simulink model "comm_test"  (R2022a)
settings: Solver=FixedStepAuto  StartTime=0.0  StopTime=20  RelTol=1e-3
libraries: hdlsllib x8, simulink x7, mbedblockslib x7
settings Model: ExtModeTrigDuration=10  Creator=FUGAZI  LastModifiedBy=FUGAZI
settings OptimizationCC: EnhancedBackFolding=on  PassReuseOutputArgsAs=Individual arguments  ZeroExternalMemoryAtStartup=off  ZeroInternalMemoryAtStartup=off  MaxStackSize=64  OptimizeBlockOrder=speed  DifferentSizesBufferReuse=on  OptimizationCustomize=off  EfficientTunableParamExpr=on
settings DebuggingCC: ParameterTunabilityLossMsg=error
settings HardwareCC: ProdBitPerPointer=32  ProdBitPerSizeT=32  ProdBitPerPtrDiffT=32  ProdLargestAtomicInteger=Long  ProdLargestAtomicFloat=Double  ProdWordSize=32  ProdLongLongMode=on  ProdHWDeviceType=ARM Compatible->ARM Cortex
settings SFSimCC: MATLABDynamicMemAlloc=off
settings RTWCC: SystemTargetFile=ert.tlc  HardwareBoard=STM32 Nucleo L476RG  TemplateMakefile=ert_default_tmf  Toolchain=GNU Tools for ARM Embedded Processors
settings CodeAppCC: ForceParamTrailComments=on  IgnoreCustomStorageClasses=off  OperatorAnnotations=on  SimulinkDataObjDesc=on  SFDataObjDesc=on  InsertBlockDesc=on
settings ERTTargetCC: ExtModeTransport=3  ExtModeStaticAlloc=on  ExtModeStaticAllocSize=2000  ExtModeMexFile=ext_xcp  ExtModeIntrfLevel=Level2 - Open

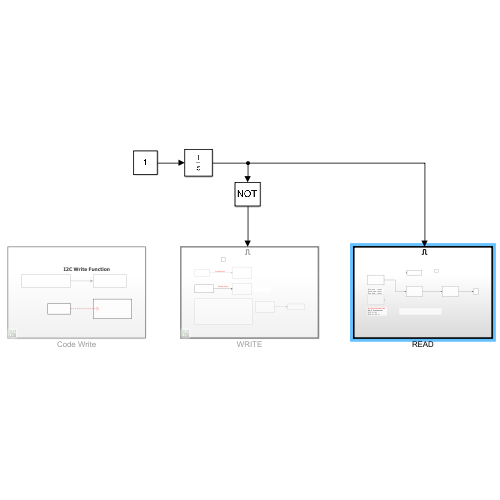
[thumbnail: Simulink's stored preview of the top-level diagram]
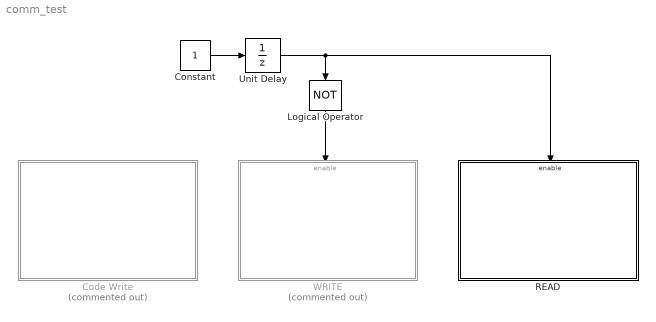
== system comm_test ==
  Code Write : Subsystem  Commented=on
  Constant : Constant  OutDataTypeStr=boolean  SampleTime=0.1
  Logical Operator : Logic  Operator=NOT  AllPortsSameDT=off  OutDataTypeStr=boolean
  READ : Subsystem
  Unit Delay : UnitDelay  SampleTime=-1  HasFrameUpgradeWarning=on
  WRITE : Subsystem  Commented=on
  wires:
  Constant/1 -> Unit Delay/1
  Logical Operator/1 -> WRITE/Enable
  Unit Delay/1 -> READ/Enable, Logical Operator/1

== system comm_test/Code Write ==
  note: I2C Write Function
  Constant : Constant  Value=[0x10, 0x00]
  Constant1 : Constant  Commented=on  Value=[hex2dec('20'), hex2dec('51')]
  Display : Display  Commented=on
  MATLAB Function : MATLAB Function  TreatAsAtomicUnit=on
  wires:
  Constant/1 -> ?
  Constant1/1 -> Display/1

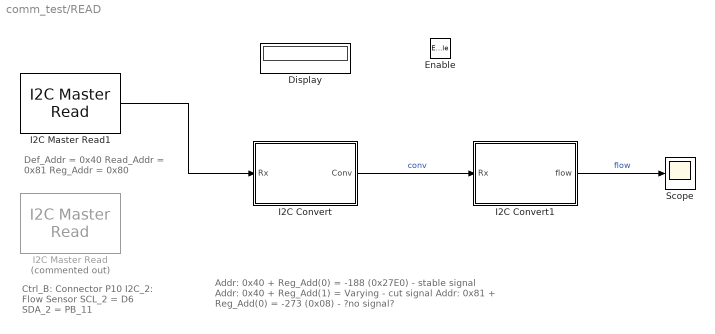
== system comm_test/READ ==
  note: Def_Addr = 0x40
      | Read_Addr = 0x81
      | Reg_Addr = 0x80
  note: Ctrl_B: Connector P10
      | I2C_2: Flow Sensor
      | SCL_2 = D6
      | SDA_2 = PB_11
  note: Addr: 0x40  + Reg_Add(0) = -188 (0x27E0) - stable signal
      | Addr: 0x40  + Reg_Add(1) = Varying            - cut signal
      | Addr: 0x81  + Reg_Add(0) = -273 (0x08)	     - ?no signal?
  Enable : EnablePort
  Display : Display
  I2C Convert : Subsystem
  I2C Convert1 : Subsystem
  I2C Master Read : mbedblockslib/I2C Master Read  Commented=on  I2CModule=0  Mode=Master  SlaveAddress=hex2dec('81')  SlaveByteOrder=BigEndian  Direction=Receiver  RegisterAddressMode=on  RegisterAddress=uint8(0)  SlaveDataType=uint8  DataLength=3  NoAck=off  RepeatedStart=on  OutputStatus=off  SampleTime=0.1
      settings: SourceProductBaseCode=MICROBIT,NUCLEO,STMICRODIS
  I2C Master Read1 : mbedblockslib/I2C Master Read  I2CModule=0  Mode=Master  SlaveAddress=hex2dec('40')  SlaveByteOrder=BigEndian  Direction=Receiver  RegisterAddressMode=off  RegisterAddress=uint8(1)  SlaveDataType=uint8  DataLength=3  NoAck=off  RepeatedStart=off  OutputStatus=off  SampleTime=0.5
      settings: SourceProductBaseCode=MICROBIT,NUCLEO,STMICRODIS
  Scope : Scope
  wires:
  I2C Convert1/1(flow) -> Scope/1  "flow"
  I2C Master Read1/1 -> I2C Convert/1(Rx)
  I2C Convert/1(Conv) -> I2C Convert1/1(Rx)  "conv"

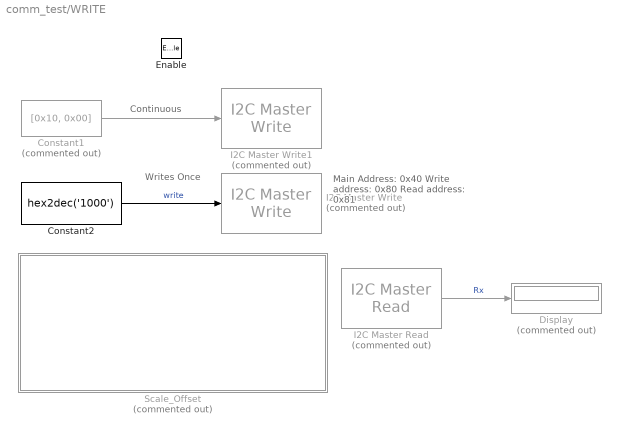
== system comm_test/WRITE ==
  note: Writes Once
  note: Main Address: 0x40
      | Write address: 0x80
      | Read address: 0x81
  note: Continuous
  Enable : EnablePort
  Constant1 : Constant  Commented=on  Value=[0x10, 0x00]
  Constant2 : Constant  Value=hex2dec('1000')  OutDataTypeStr=uint16
  Display : Display  Commented=on
  I2C Master Read : mbedblockslib/I2C Master Read  Commented=on  I2CModule=0  Mode=Master  SlaveAddress=hex2dec('40')  SlaveByteOrder=BigEndian  Direction=Receiver  RegisterAddressMode=on  RegisterAddress=uint8(1)  SlaveDataType=uint8  DataLength=3  NoAck=off  RepeatedStart=on  OutputStatus=off  SampleTime=0.1
      settings: SourceProductBaseCode=MICROBIT,NUCLEO,STMICRODIS
  I2C Master Write : mbedblockslib/I2C Master Write  Commented=on  I2CModule=0  Mode=Master  SlaveAddress=hex2dec('40')  SlaveByteOrder=BigEndian  Direction=Transmitter  RegisterAddressMode=on  RegisterAddress=uint8(1)  SlaveDataType=uint8  DataLength=2  NoAck=off  RepeatedStart=on  OutputStatus=off
      settings: SourceProductBaseCode=MICROBIT,NUCLEO,STMICRODIS
  I2C Master Write1 : mbedblockslib/I2C Master Write  Commented=on  I2CModule=0  Mode=Master  SlaveAddress=hex2dec('40')  SlaveByteOrder=BigEndian  Direction=Transmitter  RegisterAddressMode=on  RegisterAddress=uint8(1)  SlaveDataType=uint8  DataLength=2  NoAck=off  RepeatedStart=on  OutputStatus=off
      settings: SourceProductBaseCode=MICROBIT,NUCLEO,STMICRODIS
  Scale_Offset : Subsystem  Commented=on
  wires:
  Constant2/1 -> I2C Master Write/1  "write"
  Constant1/1 -> I2C Master Write1/1
  I2C Master Read/1 -> Display/1  "Rx"

== system comm_test/READ/I2C Convert ==
  note: Possible Range:
      | 0x0666 = -xx SLM
      | 0x1FF7 = 0 SLM
      | 0x3999 = xx SLM
  note: Flow Rate Range: 10sL/m - 80sL/m
  note: I2C:
      | * 1 byte @ 16-bit
      | * 2 byte @ 8-bit
      | * 3 byte @ 8-bit
      | * 4 byte @ 8-bit
  note: Add 3rd byte for CRC?
  Rx : Inport
  (2x) 8-bit : Subsystem  Commented=on
  (3x) 8-bit : Subsystem
  (4x) 8-bit : Subsystem  Commented=on
  Conv : Outport
  wires:
  Rx/1 -> (3x) 8-bit/1(Rx)  "Rx"
  (3x) 8-bit/1(3-byte) -> Conv/1  "3_byte"

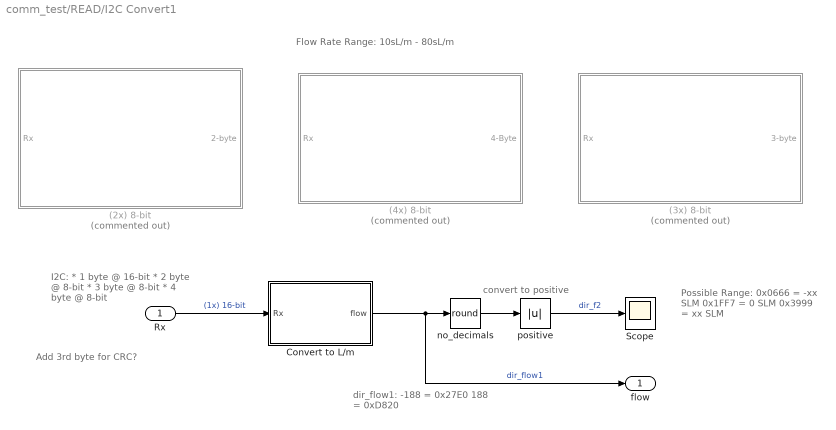
== system comm_test/READ/I2C Convert1 ==
  note: dir_flow1:
      | -188 = 0x27E0
      | 188 = 0xD820
  note: Possible Range:
      | 0x0666 = -xx SLM
      | 0x1FF7 = 0 SLM
      | 0x3999 = xx SLM
  note: Flow Rate Range: 10sL/m - 80sL/m
  note: I2C:
      | * 1 byte @ 16-bit
      | * 2 byte @ 8-bit
      | * 3 byte @ 8-bit
      | * 4 byte @ 8-bit
  note: Add 3rd byte for CRC?
  note: convert to positive
  Rx : Inport
  (2x) 8-bit : Subsystem  Commented=on
  (3x) 8-bit : Subsystem  Commented=on
  (4x) 8-bit : Subsystem  Commented=on
  Convert to L/m : Subsystem
  Scope : Scope
  no_decimals : Rounding  Operator=round
  positive : Abs  SaturateOnIntegerOverflow=off
  flow : Outport
  wires:
  Convert to L/m/1(flow) -> flow/1, no_decimals/1  "dir_flow1"
  no_decimals/1 -> positive/1
  Rx/1 -> Convert to L/m/1(Rx)  "(1x) 16-bit"
  positive/1 -> Scope/1  "dir_f2"

== system comm_test/WRITE/Scale_Offset ==
  note: Should be ~0.5ms between writes
  Constant3 : Constant  Value=[hex2dec('31E3'), hex2dec('31E4')]  OutDataTypeStr=uint16
  Display : Display  Commented=on
      settings: Format=hex (Stored Integer)
  Display1 : Display
      settings: Format=hex (Stored Integer)
  I2C Master Read : mbedblockslib/I2C Master Read  I2CModule=0  Mode=Master  SlaveAddress=hex2dec('40')  SlaveByteOrder=BigEndian  Direction=Receiver  RegisterAddressMode=on  RegisterAddress=uint8(1)  SlaveDataType=uint16  DataLength=1  NoAck=off  RepeatedStart=off  OutputStatus=off  SampleTime=0.1
      settings: SourceProductBaseCode=MICROBIT,NUCLEO,STMICRODIS
  I2C Master Write2 : mbedblockslib/I2C Master Write  I2CModule=0  Mode=Master  SlaveAddress=hex2dec('40')  SlaveByteOrder=BigEndian  Direction=Transmitter  RegisterAddressMode=on  RegisterAddress=uint8(1)  SlaveDataType=uint8  DataLength=2  NoAck=off  RepeatedStart=on  OutputStatus=off
      settings: SourceProductBaseCode=MICROBIT,NUCLEO,STMICRODIS
  wires:
  Constant3/1 -> I2C Master Write2/1, Display/1  "offset_scale"
  I2C Master Read/1 -> Display1/1  "read"

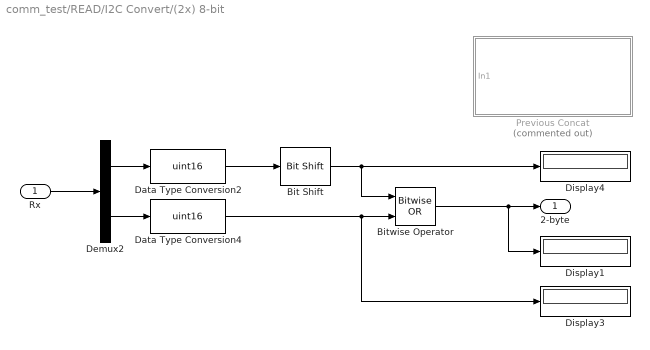
== system comm_test/READ/I2C Convert/(2x) 8-bit ==
  Rx : Inport
  Bit Shift : hdlsllib/Logic and Bit Operations/Bit Shift  mode=Shift Left Logical  N=8
  Bitwise Operator : simulink/Logic and Bit Operations/Bitwise Operator  logicop=OR  UseBitMask=off  NumInputPorts=2  BitMask=bin2dec('11011001')  BitMaskRealWorld=Stored Integer
  Data Type Conversion2 : DataTypeConversion  OutDataTypeStr=uint16  SaturateOnIntegerOverflow=off  RndMeth=Floor
  Data Type Conversion4 : DataTypeConversion  OutDataTypeStr=uint16  SaturateOnIntegerOverflow=off  RndMeth=Floor
  Demux2 : Demux  Outputs=2
  Display1 : Display
      settings: Format=hex (Stored Integer)
  Display3 : Display
      settings: Format=hex (Stored Integer)
  Display4 : Display
      settings: Format=hex (Stored Integer)
  Previous Concat : Subsystem  Commented=on
  2-byte : Outport
  wires:
  Rx/1 -> Demux2/1
  Demux2/1 -> Data Type Conversion2/1
  Data Type Conversion2/1 -> Bit Shift/1
  Bit Shift/1 -> Display4/1, Bitwise Operator/1
  Data Type Conversion4/1 -> Display3/1, Bitwise Operator/2
  Demux2/2 -> Data Type Conversion4/1
  Bitwise Operator/1 -> Display1/1, 2-byte/1

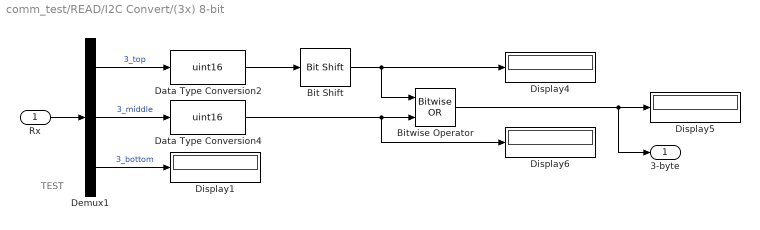
== system comm_test/READ/I2C Convert/(3x) 8-bit ==
  note: TEST
  Rx : Inport
  Bit Shift : hdlsllib/Logic and Bit Operations/Bit Shift  mode=Shift Left Logical  N=8
  Bitwise Operator : simulink/Logic and Bit Operations/Bitwise Operator  logicop=OR  UseBitMask=off  NumInputPorts=2  BitMask=bin2dec('11011001')  BitMaskRealWorld=Stored Integer
  Data Type Conversion2 : DataTypeConversion  OutDataTypeStr=uint16  SaturateOnIntegerOverflow=off  RndMeth=Floor
  Data Type Conversion4 : DataTypeConversion  OutDataTypeStr=uint16  SaturateOnIntegerOverflow=off  RndMeth=Floor
  Demux1 : Demux  Outputs=3
  Display{1,4..6} (4 alike) : Display
      settings: Format=hex (Stored Integer)
  3-byte : Outport
  wires:
  Bit Shift/1 -> Bitwise Operator/1, Display4/1
  Data Type Conversion4/1 -> Display6/1, Bitwise Operator/2
  Bitwise Operator/1 -> 3-byte/1, Display5/1
  Data Type Conversion2/1 -> Bit Shift/1
  Rx/1 -> Demux1/1
  Demux1/1 -> Data Type Conversion2/1  "3_top"
  Demux1/2 -> Data Type Conversion4/1  "3_middle"
  Demux1/3 -> Display1/1  "3_bottom"

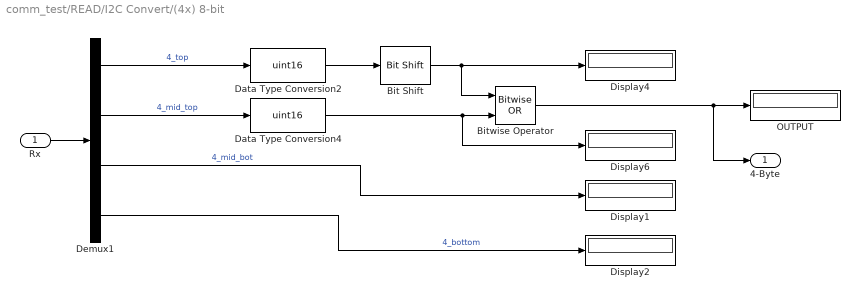
== system comm_test/READ/I2C Convert/(4x) 8-bit ==
  Rx : Inport
  Bit Shift : hdlsllib/Logic and Bit Operations/Bit Shift  mode=Shift Left Logical  N=8
  Bitwise Operator : simulink/Logic and Bit Operations/Bitwise Operator  logicop=OR  UseBitMask=off  NumInputPorts=2  BitMask=bin2dec('11011001')  BitMaskRealWorld=Stored Integer
  Data Type Conversion2 : DataTypeConversion  OutDataTypeStr=uint16  SaturateOnIntegerOverflow=off  RndMeth=Floor
  Data Type Conversion4 : DataTypeConversion  OutDataTypeStr=uint16  SaturateOnIntegerOverflow=off  RndMeth=Floor
  Demux1 : Demux
  Display{1..2,4,6} (4 alike) : Display
      settings: Format=hex (Stored Integer)
  OUTPUT : Display
      settings: Format=hex (Stored Integer)
  4-Byte : Outport
  wires:
  Data Type Conversion2/1 -> Bit Shift/1
  Bitwise Operator/1 -> 4-Byte/1, OUTPUT/1
  Bit Shift/1 -> Display4/1, Bitwise Operator/1
  Demux1/4 -> Display2/1  "4_bottom"
  Rx/1 -> Demux1/1
  Demux1/2 -> Data Type Conversion4/1  "4_mid_top"
  Demux1/1 -> Data Type Conversion2/1  "4_top"
  Data Type Conversion4/1 -> Display6/1, Bitwise Operator/2
  Demux1/3 -> Display1/1  "4_mid_bot"

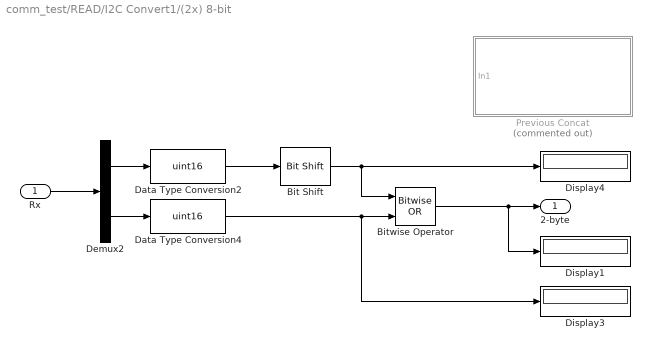
== system comm_test/READ/I2C Convert1/(2x) 8-bit ==
  Rx : Inport
  Bit Shift : hdlsllib/Logic and Bit Operations/Bit Shift  mode=Shift Left Logical  N=8
  Bitwise Operator : simulink/Logic and Bit Operations/Bitwise Operator  logicop=OR  UseBitMask=off  NumInputPorts=2  BitMask=bin2dec('11011001')  BitMaskRealWorld=Stored Integer
  Data Type Conversion2 : DataTypeConversion  OutDataTypeStr=uint16  SaturateOnIntegerOverflow=off  RndMeth=Floor
  Data Type Conversion4 : DataTypeConversion  OutDataTypeStr=uint16  SaturateOnIntegerOverflow=off  RndMeth=Floor
  Demux2 : Demux  Outputs=2
  Display1 : Display
      settings: Format=hex (Stored Integer)
  Display3 : Display
      settings: Format=hex (Stored Integer)
  Display4 : Display
      settings: Format=hex (Stored Integer)
  Previous Concat : Subsystem  Commented=on
  2-byte : Outport
  wires:
  Rx/1 -> Demux2/1
  Demux2/1 -> Data Type Conversion2/1
  Data Type Conversion2/1 -> Bit Shift/1
  Bit Shift/1 -> Display4/1, Bitwise Operator/1
  Data Type Conversion4/1 -> Display3/1, Bitwise Operator/2
  Demux2/2 -> Data Type Conversion4/1
  Bitwise Operator/1 -> Display1/1, 2-byte/1

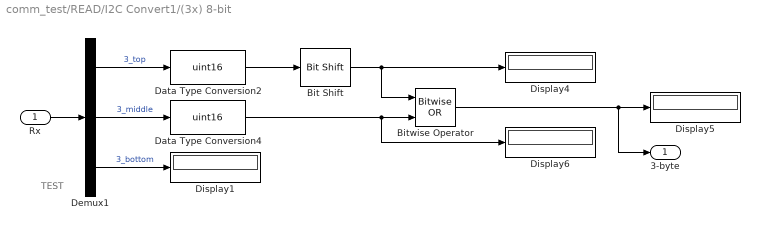
== system comm_test/READ/I2C Convert1/(3x) 8-bit ==
  note: TEST
  Rx : Inport
  Bit Shift : hdlsllib/Logic and Bit Operations/Bit Shift  mode=Shift Left Logical  N=8
  Bitwise Operator : simulink/Logic and Bit Operations/Bitwise Operator  logicop=OR  UseBitMask=off  NumInputPorts=2  BitMask=bin2dec('11011001')  BitMaskRealWorld=Stored Integer
  Data Type Conversion2 : DataTypeConversion  OutDataTypeStr=uint16  SaturateOnIntegerOverflow=off  RndMeth=Floor
  Data Type Conversion4 : DataTypeConversion  OutDataTypeStr=uint16  SaturateOnIntegerOverflow=off  RndMeth=Floor
  Demux1 : Demux  Outputs=3
  Display{1,4..6} (4 alike) : Display
      settings: Format=hex (Stored Integer)
  3-byte : Outport
  wires:
  Bit Shift/1 -> Bitwise Operator/1, Display4/1
  Data Type Conversion4/1 -> Display6/1, Bitwise Operator/2
  Bitwise Operator/1 -> 3-byte/1, Display5/1
  Data Type Conversion2/1 -> Bit Shift/1
  Rx/1 -> Demux1/1
  Demux1/1 -> Data Type Conversion2/1  "3_top"
  Demux1/2 -> Data Type Conversion4/1  "3_middle"
  Demux1/3 -> Display1/1  "3_bottom"

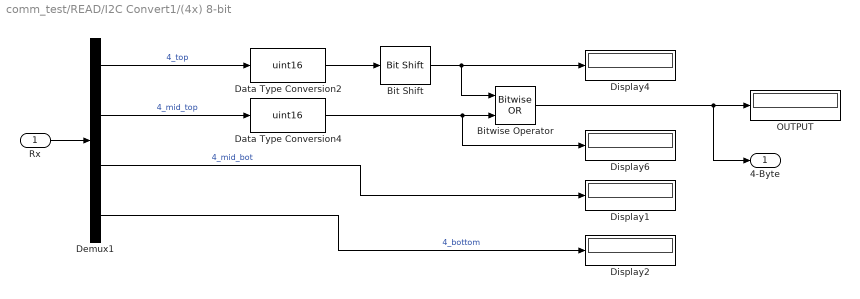
== system comm_test/READ/I2C Convert1/(4x) 8-bit ==
  Rx : Inport
  Bit Shift : hdlsllib/Logic and Bit Operations/Bit Shift  mode=Shift Left Logical  N=8
  Bitwise Operator : simulink/Logic and Bit Operations/Bitwise Operator  logicop=OR  UseBitMask=off  NumInputPorts=2  BitMask=bin2dec('11011001')  BitMaskRealWorld=Stored Integer
  Data Type Conversion2 : DataTypeConversion  OutDataTypeStr=uint16  SaturateOnIntegerOverflow=off  RndMeth=Floor
  Data Type Conversion4 : DataTypeConversion  OutDataTypeStr=uint16  SaturateOnIntegerOverflow=off  RndMeth=Floor
  Demux1 : Demux
  Display{1..2,4,6} (4 alike) : Display
      settings: Format=hex (Stored Integer)
  OUTPUT : Display
      settings: Format=hex (Stored Integer)
  4-Byte : Outport
  wires:
  Data Type Conversion2/1 -> Bit Shift/1
  Bitwise Operator/1 -> 4-Byte/1, OUTPUT/1
  Bit Shift/1 -> Display4/1, Bitwise Operator/1
  Demux1/4 -> Display2/1  "4_bottom"
  Rx/1 -> Demux1/1
  Demux1/2 -> Data Type Conversion4/1  "4_mid_top"
  Demux1/1 -> Data Type Conversion2/1  "4_top"
  Data Type Conversion4/1 -> Display6/1, Bitwise Operator/2
  Demux1/3 -> Display1/1  "4_mid_bot"

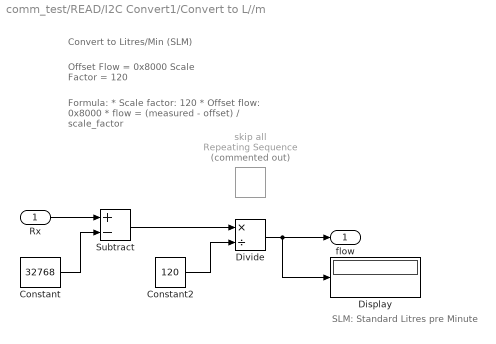
== system comm_test/READ/I2C Convert1/Convert to L//m ==
  note: SLM: Standard Litres pre Minute
  note: Convert to Litres/Min (SLM)
  note: Offset Flow = 0x8000
      | Scale Factor = 120
  note: Formula:
      | * Scale factor: 120
      | * Offset flow: 0x8000
      | * flow = (measured - offset) / scale_factor
  Rx : Inport
  Constant : Constant  Value=32768
  Constant2 : Constant  Value=120
  Display : Display
  Divide : Product  Inputs=*/
  Subtract : Sum  Inputs=+-
  skip all : simulink/Sources/Repeating Sequence  Commented=on  rep_seq_t=[0 1.3 1.31 2.5 2.51]  rep_seq_y=[30 30 150 150 30]
  flow : Outport
  wires:
  Divide/1 -> Display/1, flow/1
  Subtract/1 -> Divide/1
  Constant2/1 -> Divide/2
  Constant/1 -> Subtract/2
  Rx/1 -> Subtract/1

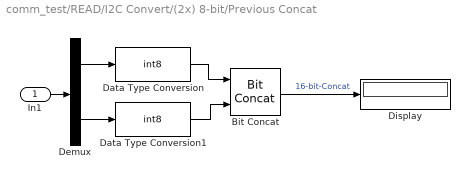
== system comm_test/READ/I2C Convert/(2x) 8-bit/Previous Concat ==
  In1 : Inport
  Bit Concat : hdlsllib/Logic and Bit Operations/Bit Concat  numInputs=2
  Data Type Conversion : DataTypeConversion  OutDataTypeStr=int8  SaturateOnIntegerOverflow=off  RndMeth=Floor
  Data Type Conversion1 : DataTypeConversion  OutDataTypeStr=int8  SaturateOnIntegerOverflow=off  RndMeth=Floor
  Demux : Demux  Outputs=2
  Display : Display
      settings: Format=hex (Stored Integer)
  wires:
  Data Type Conversion/1 -> Bit Concat/1
  Bit Concat/1 -> Display/1  "16-bit-Concat"
  Demux/2 -> Data Type Conversion1/1
  Data Type Conversion1/1 -> Bit Concat/2
  Demux/1 -> Data Type Conversion/1
  In1/1 -> Demux/1

== system comm_test/READ/I2C Convert1/(2x) 8-bit/Previous Concat ==
  In1 : Inport
  Bit Concat : hdlsllib/Logic and Bit Operations/Bit Concat  numInputs=2
  Data Type Conversion : DataTypeConversion  OutDataTypeStr=int8  SaturateOnIntegerOverflow=off  RndMeth=Floor
  Data Type Conversion1 : DataTypeConversion  OutDataTypeStr=int8  SaturateOnIntegerOverflow=off  RndMeth=Floor
  Demux : Demux  Outputs=2
  Display : Display
      settings: Format=hex (Stored Integer)
  wires:
  Data Type Conversion/1 -> Bit Concat/1
  Bit Concat/1 -> Display/1  "16-bit-Concat"
  Demux/2 -> Data Type Conversion1/1
  Data Type Conversion1/1 -> Bit Concat/2
  Demux/1 -> Data Type Conversion/1
  In1/1 -> Demux/1

== matlab function comm_test/Code Write/MATLAB Function ==
function writeByteToSTM32()
    % Constants
    deviceAddress = uint8(hex2dec('40'));
    byteToWrite = uint8(hex2dec('10'));
    port = 'COM4';

    % Create serial object
    s = serialport(port, 'BaudRate', 9600);
    
    % Open the serial connection
    fopen(s);

    % Send command to switch to I2C mode
    fprintf(s, 'I2C_MODE');

    % Wait for the device to be ready
    pause(0.1);

    % Send the write command, followed by the device address and the byte to write
    fprintf(s, 'I2C_WRITE');
    fwrite(s, deviceAddress);
    fwrite(s, byteToWrite);

    % Close the serial connection
    fclose(s);

    % Delete the serial object
    delete(s);
end
